simulink model "secondEquationSystem"  (R2024a)
settings: Solver=VariableStepAuto  StartTime=0.0  StopTime=10.0  RelTol=1e-3
settings Model: Creator=andrey  LastModifiedBy=andrey

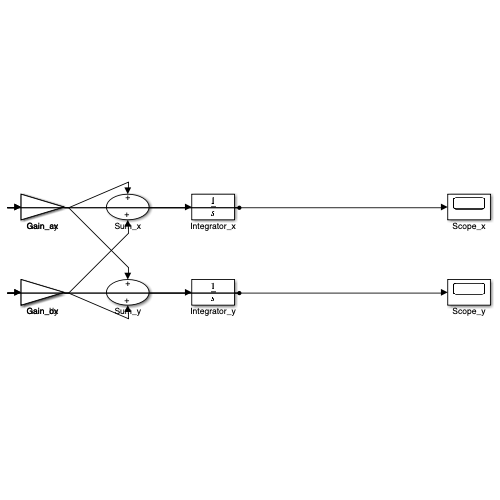
[thumbnail: Simulink's stored preview of the top-level diagram]
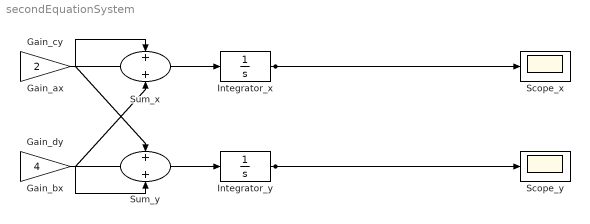
== system secondEquationSystem ==
  Gain_ax : Gain  Gain=3
  Gain_bx : Gain  Gain=3
  Gain_cy : Gain  Gain=2
  Gain_dy : Gain  Gain=4
  Integrator_x : Integrator
  Integrator_y : Integrator
  Scope_x : Scope
  Scope_y : Scope
  Sum_x : Sum
  Sum_y : Sum
  wires:
  Sum_x/1 -> Integrator_x/1
  Sum_y/1 -> Integrator_y/1
  Integrator_x/1 -> Scope_x/1, Gain_ax/1, Gain_cy/1
  Integrator_y/1 -> Scope_y/1, Gain_bx/1, Gain_dy/1
  Gain_ax/1 -> Sum_x/1
  Gain_bx/1 -> Sum_x/2
  Gain_cy/1 -> Sum_y/1
  Gain_dy/1 -> Sum_y/2
